simulink model "MdXX_DoneChk"  (R2024b)
settings: Solver=FixedStepDiscrete  StartTime=0.0  StopTime=10.0  FixedStep=0.01  RelTol=1e-3
undefined symbols (not defined in the file or in its folder): KeSMSuVehicleModelConfig_Val
libraries: simulink x44
(part 2 of 3)

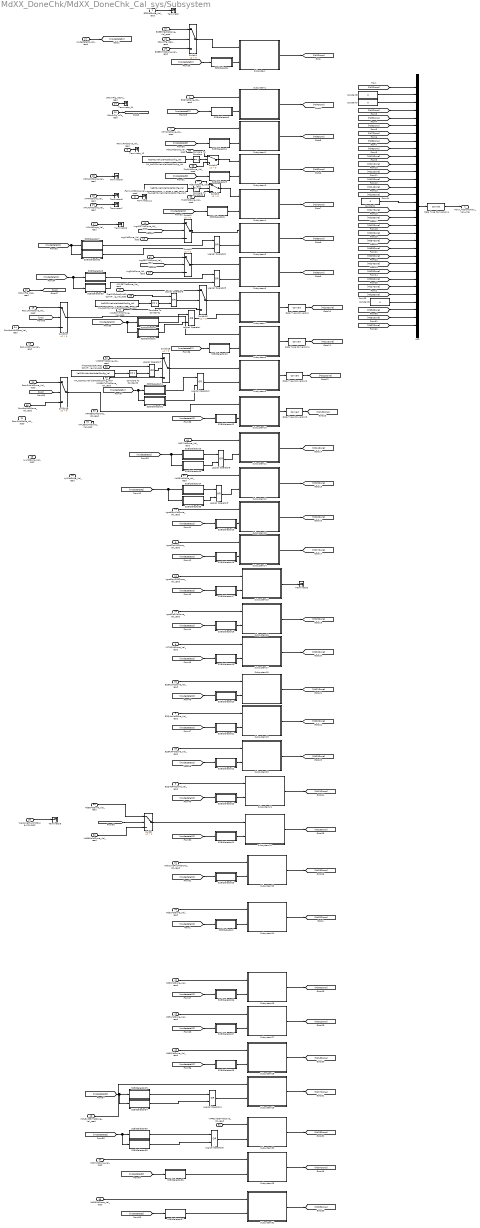
== system MdXX_DoneChk/MdXX_DoneChk_Cal_sys/Subsystem ==
  EZEMdDone_Val_read : Inport
  EZQ4sLMdDone_Val_read : Inport  Port=2
  EZQ4sRMdDone_Val_read : Inport  Port=3
  EZQMdDone_Val_read : Inport  Port=4
  FamlyLMdDone_Val_read : Inport  Port=5
  FamlyRMdDone_Val_read : Inport  Port=6
  INTMLMdDone_Val_read : Inport  Port=7
  INTMRMdDone_Val_read : Inport  Port=8
  LgrstClsLMdDone_Val_read : Inport  Port=9
  LgrstClsRMdDone_Val_read : Inport  Port=10
  LgrstOpnLMdDone_Val_read : Inport  Port=11
  LgrstOpnRMdDone_Val_read : Inport  Port=12
  LugLMdDone_Val_read : Inport  Port=13
  LugRMdDone_Val_read : Inport  Port=14
  LyLMdDone_Val_read : Inport  Port=15
  LyRMdDone_Val_read : Inport  Port=16
  modestate32_Val_read : Inport  Port=17
  RecvL4sMdDone_Val_read : Inport  Port=18
  RecvLMdDone_Val_read : Inport  Port=19
  RecvR4sMdDone_Val_read : Inport  Port=20
  RecvRMdDone_Val_read : Inport  Port=21
  StNumFlg_Is4s_read : Inport  Port=22
  StNumFlg_Is6s_read : Inport  Port=23
  StNumFlg_Is6s7s_read : Inport  Port=24
  StNumFlg_Is7s_read : Inport  Port=25
  VIPL4sMdDone_Val_read : Inport  Port=26
  VIPLMdDone_Val_read : Inport  Port=27
  VIPR4sMdDone_Val_read : Inport  Port=28
  VIPRMdDone_Val_read : Inport  Port=29
  WelcomeBkwdMdDone_Val_read : Inport  Port=30
  WelcomeFwdMdDone_Val_read : Inport  Port=31
  EZE4sLMdDone_Val_read : Inport  Port=32
  EZE4sRMdDone_Val_read : Inport  Port=33
  ComfortMdLDone_Val_read : Inport  Port=34
  ComfortMdRDone_Val_read : Inport  Port=35
  EZE557MdDone_Val_read : Inport  Port=36
  EZE5576sMdDone_Val_read : Inport  Port=37
  IfVeSMSbSecRwLtStCshnFrntUpwdDnwdMovConfig_Val_read : Inport  Port=38
  IfVeSMSbSecRwRtStCshnFrntUpwdDnwdMovConfig_Val_read : Inport  Port=39
  LugL557MdDone_Val_read : Inport  Port=40
  LugR557MdDone_Val_read : Inport  Port=41
  Md30MdDone_Val_read : Inport  Port=42
  Md31MdDone_Val_read : Inport  Port=43
  Md32MdDone_Val_read : Inport  Port=44
  Md53MdDone_Val_read : Inport  Port=45
  VIPL557LTMdDone_Val_read : Inport  Port=46
  VIPL557MdDone_Val_read : Inport  Port=47
  VIPLExit557MdDone_Val_read : Inport  Port=48
  VIPR557LTMdDone_Val_read : Inport  Port=49
  VIPR557MdDone_Val_read : Inport  Port=50
  VIPRExit557MdDone_Val_read : Inport  Port=51
  Md566sMdDone_Val_read : Inport  Port=52
  Md56MdDone_Val_read : Inport  Port=53
  Md57MdDone_Val_read : Inport  Port=54
  Md58MdDone_Val_read : Inport  Port=55
  Md61MdDone_Val_read : Inport  Port=56
  Md62MdDone_Val_read : Inport  Port=57
  FwdLMdDone_Val_read : Inport  Port=58
  FwdRMdDone_Val_read : Inport  Port=59
  Md27MdDone_Val_read : Inport  Port=60
  Md28MdDone_Val_read : Inport  Port=61
  VIPL3582MdDone_Val_read : Inport  Port=62
  VIPR3582MdDone_Val_read : Inport  Port=63
  32BitSelector : Subsystem  mask(32 Bit Selector){BitNum=0}
      mask prompts: BitNum "Select Bit Number"
      mask help: Allows selection of a particular bit (0-31) out of a packed word up to 32 bits long. Output will be true if the bit number selected via the mask parameter is equal to one.
      mask TypeOptions BitNum: 0 | 1 | 2 | 3 | 4 | 5 | 6 | 7 | 8 | 9 | 10 | 11 | 12 | 13 | 14 | 15 | 16 | 17 | 18 | 19 | 20 | 21 | 22 | 23 | 24 | 25 | 26 | 27 | 28 | 29 | 30 | 31
      mask Display:
      | text(0.5, 0.8,'BIT','horizontalAlignment','center')
      | text(0.5, 0.5,'SELECTOR','horizontalAlignment','center')
      | text(0.5, 0.2,['-- Bit ',char(get_param(gcb,'BitNum')),' --'],'horizontalAlignment','center')
  32BitSelector1 : Subsystem  mask(32 Bit Selector){BitNum=31}
      mask prompts: BitNum "Select Bit Number"
      mask help: Allows selection of a particular bit (0-31) out of a packed word up to 32 bits long. Output will be true if the bit number selected via the mask parameter is equal to one.
      mask TypeOptions BitNum: 0 | 1 | 2 | 3 | 4 | 5 | 6 | 7 | 8 | 9 | 10 | 11 | 12 | 13 | 14 | 15 | 16 | 17 | 18 | 19 | 20 | 21 | 22 | 23 | 24 | 25 | 26 | 27 | 28 | 29 | 30 | 31
      mask Display:
      | text(0.5, 0.8,'BIT','horizontalAlignment','center')
      | text(0.5, 0.5,'SELECTOR','horizontalAlignment','center')
      | text(0.5, 0.2,['-- Bit ',char(get_param(gcb,'BitNum')),' --'],'horizontalAlignment','center')
  32BitSelector10 : Subsystem  mask(32 Bit Selector){BitNum=10}
      mask prompts: BitNum "Select Bit Number"
      mask help: Allows selection of a particular bit (0-31) out of a packed word up to 32 bits long. Output will be true if the bit number selected via the mask parameter is equal to one.
      mask TypeOptions BitNum: 0 | 1 | 2 | 3 | 4 | 5 | 6 | 7 | 8 | 9 | 10 | 11 | 12 | 13 | 14 | 15 | 16 | 17 | 18 | 19 | 20 | 21 | 22 | 23 | 24 | 25 | 26 | 27 | 28 | 29 | 30 | 31
      mask Display:
      | text(0.5, 0.8,'BIT','horizontalAlignment','center')
      | text(0.5, 0.5,'SELECTOR','horizontalAlignment','center')
      | text(0.5, 0.2,['-- Bit ',char(get_param(gcb,'BitNum')),' --'],'horizontalAlignment','center')
  32BitSelector11 : Subsystem  mask(32 Bit Selector){BitNum=11}
      mask prompts: BitNum "Select Bit Number"
      mask help: Allows selection of a particular bit (0-31) out of a packed word up to 32 bits long. Output will be true if the bit number selected via the mask parameter is equal to one.
      mask TypeOptions BitNum: 0 | 1 | 2 | 3 | 4 | 5 | 6 | 7 | 8 | 9 | 10 | 11 | 12 | 13 | 14 | 15 | 16 | 17 | 18 | 19 | 20 | 21 | 22 | 23 | 24 | 25 | 26 | 27 | 28 | 29 | 30 | 31
      mask Display:
      | text(0.5, 0.8,'BIT','horizontalAlignment','center')
      | text(0.5, 0.5,'SELECTOR','horizontalAlignment','center')
      | text(0.5, 0.2,['-- Bit ',char(get_param(gcb,'BitNum')),' --'],'horizontalAlignment','center')
  32BitSelector12 : Subsystem  mask(32 Bit Selector){BitNum=12}
      mask prompts: BitNum "Select Bit Number"
      mask help: Allows selection of a particular bit (0-31) out of a packed word up to 32 bits long. Output will be true if the bit number selected via the mask parameter is equal to one.
      mask TypeOptions BitNum: 0 | 1 | 2 | 3 | 4 | 5 | 6 | 7 | 8 | 9 | 10 | 11 | 12 | 13 | 14 | 15 | 16 | 17 | 18 | 19 | 20 | 21 | 22 | 23 | 24 | 25 | 26 | 27 | 28 | 29 | 30 | 31
      mask Display:
      | text(0.5, 0.8,'BIT','horizontalAlignment','center')
      | text(0.5, 0.5,'SELECTOR','horizontalAlignment','center')
      | text(0.5, 0.2,['-- Bit ',char(get_param(gcb,'BitNum')),' --'],'horizontalAlignment','center')
  32BitSelector13 : Subsystem  mask(32 Bit Selector){BitNum=13}
      mask prompts: BitNum "Select Bit Number"
      mask help: Allows selection of a particular bit (0-31) out of a packed word up to 32 bits long. Output will be true if the bit number selected via the mask parameter is equal to one.
      mask TypeOptions BitNum: 0 | 1 | 2 | 3 | 4 | 5 | 6 | 7 | 8 | 9 | 10 | 11 | 12 | 13 | 14 | 15 | 16 | 17 | 18 | 19 | 20 | 21 | 22 | 23 | 24 | 25 | 26 | 27 | 28 | 29 | 30 | 31
      mask Display:
      | text(0.5, 0.8,'BIT','horizontalAlignment','center')
      | text(0.5, 0.5,'SELECTOR','horizontalAlignment','center')
      | text(0.5, 0.2,['-- Bit ',char(get_param(gcb,'BitNum')),' --'],'horizontalAlignment','center')
  32BitSelector14 : Subsystem  mask(32 Bit Selector){BitNum=14}
      mask prompts: BitNum "Select Bit Number"
      mask help: Allows selection of a particular bit (0-31) out of a packed word up to 32 bits long. Output will be true if the bit number selected via the mask parameter is equal to one.
      mask TypeOptions BitNum: 0 | 1 | 2 | 3 | 4 | 5 | 6 | 7 | 8 | 9 | 10 | 11 | 12 | 13 | 14 | 15 | 16 | 17 | 18 | 19 | 20 | 21 | 22 | 23 | 24 | 25 | 26 | 27 | 28 | 29 | 30 | 31
      mask Display:
      | text(0.5, 0.8,'BIT','horizontalAlignment','center')
      | text(0.5, 0.5,'SELECTOR','horizontalAlignment','center')
      | text(0.5, 0.2,['-- Bit ',char(get_param(gcb,'BitNum')),' --'],'horizontalAlignment','center')
  32BitSelector15 : Subsystem  mask(32 Bit Selector){BitNum=15}
      mask prompts: BitNum "Select Bit Number"
      mask help: Allows selection of a particular bit (0-31) out of a packed word up to 32 bits long. Output will be true if the bit number selected via the mask parameter is equal to one.
      mask TypeOptions BitNum: 0 | 1 | 2 | 3 | 4 | 5 | 6 | 7 | 8 | 9 | 10 | 11 | 12 | 13 | 14 | 15 | 16 | 17 | 18 | 19 | 20 | 21 | 22 | 23 | 24 | 25 | 26 | 27 | 28 | 29 | 30 | 31
      mask Display:
      | text(0.5, 0.8,'BIT','horizontalAlignment','center')
      | text(0.5, 0.5,'SELECTOR','horizontalAlignment','center')
      | text(0.5, 0.2,['-- Bit ',char(get_param(gcb,'BitNum')),' --'],'horizontalAlignment','center')
  32BitSelector16 : Subsystem  mask(32 Bit Selector){BitNum=16}
      mask prompts: BitNum "Select Bit Number"
      mask help: Allows selection of a particular bit (0-31) out of a packed word up to 32 bits long. Output will be true if the bit number selected via the mask parameter is equal to one.
      mask TypeOptions BitNum: 0 | 1 | 2 | 3 | 4 | 5 | 6 | 7 | 8 | 9 | 10 | 11 | 12 | 13 | 14 | 15 | 16 | 17 | 18 | 19 | 20 | 21 | 22 | 23 | 24 | 25 | 26 | 27 | 28 | 29 | 30 | 31
      mask Display:
      | text(0.5, 0.8,'BIT','horizontalAlignment','center')
      | text(0.5, 0.5,'SELECTOR','horizontalAlignment','center')
      | text(0.5, 0.2,['-- Bit ',char(get_param(gcb,'BitNum')),' --'],'horizontalAlignment','center')
  32BitSelector17 : Subsystem  mask(32 Bit Selector){BitNum=17}
      mask prompts: BitNum "Select Bit Number"
      mask help: Allows selection of a particular bit (0-31) out of a packed word up to 32 bits long. Output will be true if the bit number selected via the mask parameter is equal to one.
      mask TypeOptions BitNum: 0 | 1 | 2 | 3 | 4 | 5 | 6 | 7 | 8 | 9 | 10 | 11 | 12 | 13 | 14 | 15 | 16 | 17 | 18 | 19 | 20 | 21 | 22 | 23 | 24 | 25 | 26 | 27 | 28 | 29 | 30 | 31
      mask Display:
      | text(0.5, 0.8,'BIT','horizontalAlignment','center')
      | text(0.5, 0.5,'SELECTOR','horizontalAlignment','center')
      | text(0.5, 0.2,['-- Bit ',char(get_param(gcb,'BitNum')),' --'],'horizontalAlignment','center')
  32BitSelector18 : Subsystem  mask(32 Bit Selector){BitNum=18}
      mask prompts: BitNum "Select Bit Number"
      mask help: Allows selection of a particular bit (0-31) out of a packed word up to 32 bits long. Output will be true if the bit number selected via the mask parameter is equal to one.
      mask TypeOptions BitNum: 0 | 1 | 2 | 3 | 4 | 5 | 6 | 7 | 8 | 9 | 10 | 11 | 12 | 13 | 14 | 15 | 16 | 17 | 18 | 19 | 20 | 21 | 22 | 23 | 24 | 25 | 26 | 27 | 28 | 29 | 30 | 31
      mask Display:
      | text(0.5, 0.8,'BIT','horizontalAlignment','center')
      | text(0.5, 0.5,'SELECTOR','horizontalAlignment','center')
      | text(0.5, 0.2,['-- Bit ',char(get_param(gcb,'BitNum')),' --'],'horizontalAlignment','center')
  32BitSelector19 : Subsystem  mask(32 Bit Selector){BitNum=19}
      mask prompts: BitNum "Select Bit Number"
      mask help: Allows selection of a particular bit (0-31) out of a packed word up to 32 bits long. Output will be true if the bit number selected via the mask parameter is equal to one.
      mask TypeOptions BitNum: 0 | 1 | 2 | 3 | 4 | 5 | 6 | 7 | 8 | 9 | 10 | 11 | 12 | 13 | 14 | 15 | 16 | 17 | 18 | 19 | 20 | 21 | 22 | 23 | 24 | 25 | 26 | 27 | 28 | 29 | 30 | 31
      mask Display:
      | text(0.5, 0.8,'BIT','horizontalAlignment','center')
      | text(0.5, 0.5,'SELECTOR','horizontalAlignment','center')
      | text(0.5, 0.2,['-- Bit ',char(get_param(gcb,'BitNum')),' --'],'horizontalAlignment','center')
  32BitSelector2 : Subsystem  mask(32 Bit Selector){BitNum=1}
      mask prompts: BitNum "Select Bit Number"
      mask help: Allows selection of a particular bit (0-31) out of a packed word up to 32 bits long. Output will be true if the bit number selected via the mask parameter is equal to one.
      mask TypeOptions BitNum: 0 | 1 | 2 | 3 | 4 | 5 | 6 | 7 | 8 | 9 | 10 | 11 | 12 | 13 | 14 | 15 | 16 | 17 | 18 | 19 | 20 | 21 | 22 | 23 | 24 | 25 | 26 | 27 | 28 | 29 | 30 | 31
      mask Display:
      | text(0.5, 0.8,'BIT','horizontalAlignment','center')
      | text(0.5, 0.5,'SELECTOR','horizontalAlignment','center')
      | text(0.5, 0.2,['-- Bit ',char(get_param(gcb,'BitNum')),' --'],'horizontalAlignment','center')
  32BitSelector20 : Subsystem  mask(32 Bit Selector){BitNum=20}
      mask prompts: BitNum "Select Bit Number"
      mask help: Allows selection of a particular bit (0-31) out of a packed word up to 32 bits long. Output will be true if the bit number selected via the mask parameter is equal to one.
      mask TypeOptions BitNum: 0 | 1 | 2 | 3 | 4 | 5 | 6 | 7 | 8 | 9 | 10 | 11 | 12 | 13 | 14 | 15 | 16 | 17 | 18 | 19 | 20 | 21 | 22 | 23 | 24 | 25 | 26 | 27 | 28 | 29 | 30 | 31
      mask Display:
      | text(0.5, 0.8,'BIT','horizontalAlignment','center')
      | text(0.5, 0.5,'SELECTOR','horizontalAlignment','center')
      | text(0.5, 0.2,['-- Bit ',char(get_param(gcb,'BitNum')),' --'],'horizontalAlignment','center')
  32BitSelector21 : Subsystem  mask(32 Bit Selector){BitNum=21}
      mask prompts: BitNum "Select Bit Number"
      mask help: Allows selection of a particular bit (0-31) out of a packed word up to 32 bits long. Output will be true if the bit number selected via the mask parameter is equal to one.
      mask TypeOptions BitNum: 0 | 1 | 2 | 3 | 4 | 5 | 6 | 7 | 8 | 9 | 10 | 11 | 12 | 13 | 14 | 15 | 16 | 17 | 18 | 19 | 20 | 21 | 22 | 23 | 24 | 25 | 26 | 27 | 28 | 29 | 30 | 31
      mask Display:
      | text(0.5, 0.8,'BIT','horizontalAlignment','center')
      | text(0.5, 0.5,'SELECTOR','horizontalAlignment','center')
      | text(0.5, 0.2,['-- Bit ',char(get_param(gcb,'BitNum')),' --'],'horizontalAlignment','center')
  32BitSelector22 : Subsystem  mask(32 Bit Selector){BitNum=22}
      mask prompts: BitNum "Select Bit Number"
      mask help: Allows selection of a particular bit (0-31) out of a packed word up to 32 bits long. Output will be true if the bit number selected via the mask parameter is equal to one.
      mask TypeOptions BitNum: 0 | 1 | 2 | 3 | 4 | 5 | 6 | 7 | 8 | 9 | 10 | 11 | 12 | 13 | 14 | 15 | 16 | 17 | 18 | 19 | 20 | 21 | 22 | 23 | 24 | 25 | 26 | 27 | 28 | 29 | 30 | 31
      mask Display:
      | text(0.5, 0.8,'BIT','horizontalAlignment','center')
      | text(0.5, 0.5,'SELECTOR','horizontalAlignment','center')
      | text(0.5, 0.2,['-- Bit ',char(get_param(gcb,'BitNum')),' --'],'horizontalAlignment','center')
  32BitSelector23 : Subsystem  mask(32 Bit Selector){BitNum=23}
      mask prompts: BitNum "Select Bit Number"
      mask help: Allows selection of a particular bit (0-31) out of a packed word up to 32 bits long. Output will be true if the bit number selected via the mask parameter is equal to one.
      mask TypeOptions BitNum: 0 | 1 | 2 | 3 | 4 | 5 | 6 | 7 | 8 | 9 | 10 | 11 | 12 | 13 | 14 | 15 | 16 | 17 | 18 | 19 | 20 | 21 | 22 | 23 | 24 | 25 | 26 | 27 | 28 | 29 | 30 | 31
      mask Display:
      | text(0.5, 0.8,'BIT','horizontalAlignment','center')
      | text(0.5, 0.5,'SELECTOR','horizontalAlignment','center')
      | text(0.5, 0.2,['-- Bit ',char(get_param(gcb,'BitNum')),' --'],'horizontalAlignment','center')
  32BitSelector24 : Subsystem  mask(32 Bit Selector){BitNum=24}
      mask prompts: BitNum "Select Bit Number"
      mask help: Allows selection of a particular bit (0-31) out of a packed word up to 32 bits long. Output will be true if the bit number selected via the mask parameter is equal to one.
      mask TypeOptions BitNum: 0 | 1 | 2 | 3 | 4 | 5 | 6 | 7 | 8 | 9 | 10 | 11 | 12 | 13 | 14 | 15 | 16 | 17 | 18 | 19 | 20 | 21 | 22 | 23 | 24 | 25 | 26 | 27 | 28 | 29 | 30 | 31
      mask Display:
      | text(0.5, 0.8,'BIT','horizontalAlignment','center')
      | text(0.5, 0.5,'SELECTOR','horizontalAlignment','center')
      | text(0.5, 0.2,['-- Bit ',char(get_param(gcb,'BitNum')),' --'],'horizontalAlignment','center')
  32BitSelector25 : Subsystem  mask(32 Bit Selector){BitNum=25}
      mask prompts: BitNum "Select Bit Number"
      mask help: Allows selection of a particular bit (0-31) out of a packed word up to 32 bits long. Output will be true if the bit number selected via the mask parameter is equal to one.
      mask TypeOptions BitNum: 0 | 1 | 2 | 3 | 4 | 5 | 6 | 7 | 8 | 9 | 10 | 11 | 12 | 13 | 14 | 15 | 16 | 17 | 18 | 19 | 20 | 21 | 22 | 23 | 24 | 25 | 26 | 27 | 28 | 29 | 30 | 31
      mask Display:
      | text(0.5, 0.8,'BIT','horizontalAlignment','center')
      | text(0.5, 0.5,'SELECTOR','horizontalAlignment','center')
      | text(0.5, 0.2,['-- Bit ',char(get_param(gcb,'BitNum')),' --'],'horizontalAlignment','center')
  32BitSelector26 : Subsystem  mask(32 Bit Selector){BitNum=29}
      mask prompts: BitNum "Select Bit Number"
      mask help: Allows selection of a particular bit (0-31) out of a packed word up to 32 bits long. Output will be true if the bit number selected via the mask parameter is equal to one.
      mask TypeOptions BitNum: 0 | 1 | 2 | 3 | 4 | 5 | 6 | 7 | 8 | 9 | 10 | 11 | 12 | 13 | 14 | 15 | 16 | 17 | 18 | 19 | 20 | 21 | 22 | 23 | 24 | 25 | 26 | 27 | 28 | 29 | 30 | 31
      mask Display:
      | text(0.5, 0.8,'BIT','horizontalAlignment','center')
      | text(0.5, 0.5,'SELECTOR','horizontalAlignment','center')
      | text(0.5, 0.2,['-- Bit ',char(get_param(gcb,'BitNum')),' --'],'horizontalAlignment','center')
  32BitSelector27 : Subsystem  mask(32 Bit Selector){BitNum=30}
      mask prompts: BitNum "Select Bit Number"
      mask help: Allows selection of a particular bit (0-31) out of a packed word up to 32 bits long. Output will be true if the bit number selected via the mask parameter is equal to one.
      mask TypeOptions BitNum: 0 | 1 | 2 | 3 | 4 | 5 | 6 | 7 | 8 | 9 | 10 | 11 | 12 | 13 | 14 | 15 | 16 | 17 | 18 | 19 | 20 | 21 | 22 | 23 | 24 | 25 | 26 | 27 | 28 | 29 | 30 | 31
      mask Display:
      | text(0.5, 0.8,'BIT','horizontalAlignment','center')
      | text(0.5, 0.5,'SELECTOR','horizontalAlignment','center')
      | text(0.5, 0.2,['-- Bit ',char(get_param(gcb,'BitNum')),' --'],'horizontalAlignment','center')
  32BitSelector28 : Subsystem  mask(32 Bit Selector){BitNum=17}
      mask prompts: BitNum "Select Bit Number"
      mask help: Allows selection of a particular bit (0-31) out of a packed word up to 32 bits long. Output will be true if the bit number selected via the mask parameter is equal to one.
      mask TypeOptions BitNum: 0 | 1 | 2 | 3 | 4 | 5 | 6 | 7 | 8 | 9 | 10 | 11 | 12 | 13 | 14 | 15 | 16 | 17 | 18 | 19 | 20 | 21 | 22 | 23 | 24 | 25 | 26 | 27 | 28 | 29 | 30 | 31
      mask Display:
      | text(0.5, 0.8,'BIT','horizontalAlignment','center')
      | text(0.5, 0.5,'SELECTOR','horizontalAlignment','center')
      | text(0.5, 0.2,['-- Bit ',char(get_param(gcb,'BitNum')),' --'],'horizontalAlignment','center')
  32BitSelector29 : Subsystem  mask(32 Bit Selector){BitNum=26}
      mask prompts: BitNum "Select Bit Number"
      mask help: Allows selection of a particular bit (0-31) out of a packed word up to 32 bits long. Output will be true if the bit number selected via the mask parameter is equal to one.
      mask TypeOptions BitNum: 0 | 1 | 2 | 3 | 4 | 5 | 6 | 7 | 8 | 9 | 10 | 11 | 12 | 13 | 14 | 15 | 16 | 17 | 18 | 19 | 20 | 21 | 22 | 23 | 24 | 25 | 26 | 27 | 28 | 29 | 30 | 31
      mask Display:
      | text(0.5, 0.8,'BIT','horizontalAlignment','center')
      | text(0.5, 0.5,'SELECTOR','horizontalAlignment','center')
      | text(0.5, 0.2,['-- Bit ',char(get_param(gcb,'BitNum')),' --'],'horizontalAlignment','center')
  32BitSelector3 : Subsystem  mask(32 Bit Selector){BitNum=3}
      mask prompts: BitNum "Select Bit Number"
      mask help: Allows selection of a particular bit (0-31) out of a packed word up to 32 bits long. Output will be true if the bit number selected via the mask parameter is equal to one.
      mask TypeOptions BitNum: 0 | 1 | 2 | 3 | 4 | 5 | 6 | 7 | 8 | 9 | 10 | 11 | 12 | 13 | 14 | 15 | 16 | 17 | 18 | 19 | 20 | 21 | 22 | 23 | 24 | 25 | 26 | 27 | 28 | 29 | 30 | 31
      mask Display:
      | text(0.5, 0.8,'BIT','horizontalAlignment','center')
      | text(0.5, 0.5,'SELECTOR','horizontalAlignment','center')
      | text(0.5, 0.2,['-- Bit ',char(get_param(gcb,'BitNum')),' --'],'horizontalAlignment','center')
  32BitSelector30 : Subsystem  mask(32 Bit Selector){BitNum=27}
      mask prompts: BitNum "Select Bit Number"
      mask help: Allows selection of a particular bit (0-31) out of a packed word up to 32 bits long. Output will be true if the bit number selected via the mask parameter is equal to one.
      mask TypeOptions BitNum: 0 | 1 | 2 | 3 | 4 | 5 | 6 | 7 | 8 | 9 | 10 | 11 | 12 | 13 | 14 | 15 | 16 | 17 | 18 | 19 | 20 | 21 | 22 | 23 | 24 | 25 | 26 | 27 | 28 | 29 | 30 | 31
      mask Display:
      | text(0.5, 0.8,'BIT','horizontalAlignment','center')
      | text(0.5, 0.5,'SELECTOR','horizontalAlignment','center')
      | text(0.5, 0.2,['-- Bit ',char(get_param(gcb,'BitNum')),' --'],'horizontalAlignment','center')
  32BitSelector31 : Subsystem  mask(32 Bit Selector){BitNum=1}
      mask prompts: BitNum "Select Bit Number"
      mask help: Allows selection of a particular bit (0-31) out of a packed word up to 32 bits long. Output will be true if the bit number selected via the mask parameter is equal to one.
      mask TypeOptions BitNum: 0 | 1 | 2 | 3 | 4 | 5 | 6 | 7 | 8 | 9 | 10 | 11 | 12 | 13 | 14 | 15 | 16 | 17 | 18 | 19 | 20 | 21 | 22 | 23 | 24 | 25 | 26 | 27 | 28 | 29 | 30 | 31
      mask Display:
      | text(0.5, 0.8,'BIT','horizontalAlignment','center')
      | text(0.5, 0.5,'SELECTOR','horizontalAlignment','center')
      | text(0.5, 0.2,['-- Bit ',char(get_param(gcb,'BitNum')),' --'],'horizontalAlignment','center')
  32BitSelector32 : Subsystem  mask(32 Bit Selector){BitNum=2}
      mask prompts: BitNum "Select Bit Number"
      mask help: Allows selection of a particular bit (0-31) out of a packed word up to 32 bits long. Output will be true if the bit number selected via the mask parameter is equal to one.
      mask TypeOptions BitNum: 0 | 1 | 2 | 3 | 4 | 5 | 6 | 7 | 8 | 9 | 10 | 11 | 12 | 13 | 14 | 15 | 16 | 17 | 18 | 19 | 20 | 21 | 22 | 23 | 24 | 25 | 26 | 27 | 28 | 29 | 30 | 31
      mask Display:
      | text(0.5, 0.8,'BIT','horizontalAlignment','center')
      | text(0.5, 0.5,'SELECTOR','horizontalAlignment','center')
      | text(0.5, 0.2,['-- Bit ',char(get_param(gcb,'BitNum')),' --'],'horizontalAlignment','center')
  32BitSelector33 : Subsystem  mask(32 Bit Selector){BitNum=2}
      mask prompts: BitNum "Select Bit Number"
      mask help: Allows selection of a particular bit (0-31) out of a packed word up to 32 bits long. Output will be true if the bit number selected via the mask parameter is equal to one.
      mask TypeOptions BitNum: 0 | 1 | 2 | 3 | 4 | 5 | 6 | 7 | 8 | 9 | 10 | 11 | 12 | 13 | 14 | 15 | 16 | 17 | 18 | 19 | 20 | 21 | 22 | 23 | 24 | 25 | 26 | 27 | 28 | 29 | 30 | 31
      mask Display:
      | text(0.5, 0.8,'BIT','horizontalAlignment','center')
      | text(0.5, 0.5,'SELECTOR','horizontalAlignment','center')
      | text(0.5, 0.2,['-- Bit ',char(get_param(gcb,'BitNum')),' --'],'horizontalAlignment','center')
  32BitSelector34 : Subsystem  mask(32 Bit Selector){BitNum=28}
      mask prompts: BitNum "Select Bit Number"
      mask help: Allows selection of a particular bit (0-31) out of a packed word up to 32 bits long. Output will be true if the bit number selected via the mask parameter is equal to one.
      mask TypeOptions BitNum: 0 | 1 | 2 | 3 | 4 | 5 | 6 | 7 | 8 | 9 | 10 | 11 | 12 | 13 | 14 | 15 | 16 | 17 | 18 | 19 | 20 | 21 | 22 | 23 | 24 | 25 | 26 | 27 | 28 | 29 | 30 | 31
      mask Display:
      | text(0.5, 0.8,'BIT','horizontalAlignment','center')
      | text(0.5, 0.5,'SELECTOR','horizontalAlignment','center')
      | text(0.5, 0.2,['-- Bit ',char(get_param(gcb,'BitNum')),' --'],'horizontalAlignment','center')
  32BitSelector35 : Subsystem  mask(32 Bit Selector){BitNum=28}
      mask prompts: BitNum "Select Bit Number"
      mask help: Allows selection of a particular bit (0-31) out of a packed word up to 32 bits long. Output will be true if the bit number selected via the mask parameter is equal to one.
      mask TypeOptions BitNum: 0 | 1 | 2 | 3 | 4 | 5 | 6 | 7 | 8 | 9 | 10 | 11 | 12 | 13 | 14 | 15 | 16 | 17 | 18 | 19 | 20 | 21 | 22 | 23 | 24 | 25 | 26 | 27 | 28 | 29 | 30 | 31
      mask Display:
      | text(0.5, 0.8,'BIT','horizontalAlignment','center')
      | text(0.5, 0.5,'SELECTOR','horizontalAlignment','center')
      | text(0.5, 0.2,['-- Bit ',char(get_param(gcb,'BitNum')),' --'],'horizontalAlignment','center')
  32BitSelector36 : Subsystem  mask(32 Bit Selector){BitNum=20}
      mask prompts: BitNum "Select Bit Number"
      mask help: Allows selection of a particular bit (0-31) out of a packed word up to 32 bits long. Output will be true if the bit number selected via the mask parameter is equal to one.
      mask TypeOptions BitNum: 0 | 1 | 2 | 3 | 4 | 5 | 6 | 7 | 8 | 9 | 10 | 11 | 12 | 13 | 14 | 15 | 16 | 17 | 18 | 19 | 20 | 21 | 22 | 23 | 24 | 25 | 26 | 27 | 28 | 29 | 30 | 31
      mask Display:
      | text(0.5, 0.8,'BIT','horizontalAlignment','center')
      | text(0.5, 0.5,'SELECTOR','horizontalAlignment','center')
      | text(0.5, 0.2,['-- Bit ',char(get_param(gcb,'BitNum')),' --'],'horizontalAlignment','center')
  32BitSelector37 : Subsystem  mask(32 Bit Selector){BitNum=21}
      mask prompts: BitNum "Select Bit Number"
      mask help: Allows selection of a particular bit (0-31) out of a packed word up to 32 bits long. Output will be true if the bit number selected via the mask parameter is equal to one.
      mask TypeOptions BitNum: 0 | 1 | 2 | 3 | 4 | 5 | 6 | 7 | 8 | 9 | 10 | 11 | 12 | 13 | 14 | 15 | 16 | 17 | 18 | 19 | 20 | 21 | 22 | 23 | 24 | 25 | 26 | 27 | 28 | 29 | 30 | 31
      mask Display:
      | text(0.5, 0.8,'BIT','horizontalAlignment','center')
      | text(0.5, 0.5,'SELECTOR','horizontalAlignment','center')
      | text(0.5, 0.2,['-- Bit ',char(get_param(gcb,'BitNum')),' --'],'horizontalAlignment','center')
  32BitSelector38 : Subsystem  mask(32 Bit Selector){BitNum=15}
      mask prompts: BitNum "Select Bit Number"
      mask help: Allows selection of a particular bit (0-31) out of a packed word up to 32 bits long. Output will be true if the bit number selected via the mask parameter is equal to one.
      mask TypeOptions BitNum: 0 | 1 | 2 | 3 | 4 | 5 | 6 | 7 | 8 | 9 | 10 | 11 | 12 | 13 | 14 | 15 | 16 | 17 | 18 | 19 | 20 | 21 | 22 | 23 | 24 | 25 | 26 | 27 | 28 | 29 | 30 | 31
      mask Display:
      | text(0.5, 0.8,'BIT','horizontalAlignment','center')
      | text(0.5, 0.5,'SELECTOR','horizontalAlignment','center')
      | text(0.5, 0.2,['-- Bit ',char(get_param(gcb,'BitNum')),' --'],'horizontalAlignment','center')
  32BitSelector39 : Subsystem  mask(32 Bit Selector){BitNum=15}
      mask prompts: BitNum "Select Bit Number"
      mask help: Allows selection of a particular bit (0-31) out of a packed word up to 32 bits long. Output will be true if the bit number selected via the mask parameter is equal to one.
      mask TypeOptions BitNum: 0 | 1 | 2 | 3 | 4 | 5 | 6 | 7 | 8 | 9 | 10 | 11 | 12 | 13 | 14 | 15 | 16 | 17 | 18 | 19 | 20 | 21 | 22 | 23 | 24 | 25 | 26 | 27 | 28 | 29 | 30 | 31
      mask Display:
      | text(0.5, 0.8,'BIT','horizontalAlignment','center')
      | text(0.5, 0.5,'SELECTOR','horizontalAlignment','center')
      | text(0.5, 0.2,['-- Bit ',char(get_param(gcb,'BitNum')),' --'],'horizontalAlignment','center')
  32BitSelector4 : Subsystem  mask(32 Bit Selector){BitNum=4}
      mask prompts: BitNum "Select Bit Number"
      mask help: Allows selection of a particular bit (0-31) out of a packed word up to 32 bits long. Output will be true if the bit number selected via the mask parameter is equal to one.
      mask TypeOptions BitNum: 0 | 1 | 2 | 3 | 4 | 5 | 6 | 7 | 8 | 9 | 10 | 11 | 12 | 13 | 14 | 15 | 16 | 17 | 18 | 19 | 20 | 21 | 22 | 23 | 24 | 25 | 26 | 27 | 28 | 29 | 30 | 31
      mask Display:
      | text(0.5, 0.8,'BIT','horizontalAlignment','center')
      | text(0.5, 0.5,'SELECTOR','horizontalAlignment','center')
      | text(0.5, 0.2,['-- Bit ',char(get_param(gcb,'BitNum')),' --'],'horizontalAlignment','center')
  32BitSelector5 : Subsystem  mask(32 Bit Selector){BitNum=5}
      mask prompts: BitNum "Select Bit Number"
      mask help: Allows selection of a particular bit (0-31) out of a packed word up to 32 bits long. Output will be true if the bit number selected via the mask parameter is equal to one.
      mask TypeOptions BitNum: 0 | 1 | 2 | 3 | 4 | 5 | 6 | 7 | 8 | 9 | 10 | 11 | 12 | 13 | 14 | 15 | 16 | 17 | 18 | 19 | 20 | 21 | 22 | 23 | 24 | 25 | 26 | 27 | 28 | 29 | 30 | 31
      mask Display:
      | text(0.5, 0.8,'BIT','horizontalAlignment','center')
      | text(0.5, 0.5,'SELECTOR','horizontalAlignment','center')
      | text(0.5, 0.2,['-- Bit ',char(get_param(gcb,'BitNum')),' --'],'horizontalAlignment','center')
  32BitSelector6 : Subsystem  mask(32 Bit Selector){BitNum=6}
      mask prompts: BitNum "Select Bit Number"
      mask help: Allows selection of a particular bit (0-31) out of a packed word up to 32 bits long. Output will be true if the bit number selected via the mask parameter is equal to one.
      mask TypeOptions BitNum: 0 | 1 | 2 | 3 | 4 | 5 | 6 | 7 | 8 | 9 | 10 | 11 | 12 | 13 | 14 | 15 | 16 | 17 | 18 | 19 | 20 | 21 | 22 | 23 | 24 | 25 | 26 | 27 | 28 | 29 | 30 | 31
      mask Display:
      | text(0.5, 0.8,'BIT','horizontalAlignment','center')
      | text(0.5, 0.5,'SELECTOR','horizontalAlignment','center')
      | text(0.5, 0.2,['-- Bit ',char(get_param(gcb,'BitNum')),' --'],'horizontalAlignment','center')
  32BitSelector7 : Subsystem  mask(32 Bit Selector){BitNum=7}
      mask prompts: BitNum "Select Bit Number"
      mask help: Allows selection of a particular bit (0-31) out of a packed word up to 32 bits long. Output will be true if the bit number selected via the mask parameter is equal to one.
      mask TypeOptions BitNum: 0 | 1 | 2 | 3 | 4 | 5 | 6 | 7 | 8 | 9 | 10 | 11 | 12 | 13 | 14 | 15 | 16 | 17 | 18 | 19 | 20 | 21 | 22 | 23 | 24 | 25 | 26 | 27 | 28 | 29 | 30 | 31
      mask Display:
      | text(0.5, 0.8,'BIT','horizontalAlignment','center')
      | text(0.5, 0.5,'SELECTOR','horizontalAlignment','center')
      | text(0.5, 0.2,['-- Bit ',char(get_param(gcb,'BitNum')),' --'],'horizontalAlignment','center')
  32BitSelector8 : Subsystem  mask(32 Bit Selector){BitNum=8}
      mask prompts: BitNum "Select Bit Number"
      mask help: Allows selection of a particular bit (0-31) out of a packed word up to 32 bits long. Output will be true if the bit number selected via the mask parameter is equal to one.
      mask TypeOptions BitNum: 0 | 1 | 2 | 3 | 4 | 5 | 6 | 7 | 8 | 9 | 10 | 11 | 12 | 13 | 14 | 15 | 16 | 17 | 18 | 19 | 20 | 21 | 22 | 23 | 24 | 25 | 26 | 27 | 28 | 29 | 30 | 31
      mask Display:
      | text(0.5, 0.8,'BIT','horizontalAlignment','center')
      | text(0.5, 0.5,'SELECTOR','horizontalAlignment','center')
      | text(0.5, 0.2,['-- Bit ',char(get_param(gcb,'BitNum')),' --'],'horizontalAlignment','center')
  32BitSelector9 : Subsystem  mask(32 Bit Selector){BitNum=9}
      mask prompts: BitNum "Select Bit Number"
      mask help: Allows selection of a particular bit (0-31) out of a packed word up to 32 bits long. Output will be true if the bit number selected via the mask parameter is equal to one.
      mask TypeOptions BitNum: 0 | 1 | 2 | 3 | 4 | 5 | 6 | 7 | 8 | 9 | 10 | 11 | 12 | 13 | 14 | 15 | 16 | 17 | 18 | 19 | 20 | 21 | 22 | 23 | 24 | 25 | 26 | 27 | 28 | 29 | 30 | 31
      mask Display:
      | text(0.5, 0.8,'BIT','horizontalAlignment','center')
      | text(0.5, 0.5,'SELECTOR','horizontalAlignment','center')
      | text(0.5, 0.2,['-- Bit ',char(get_param(gcb,'BitNum')),' --'],'horizontalAlignment','center')
  Compare To Constant{,1..3} (4 alike) : simulink/Logic and Bit Operations/Compare To Constant  relop===  const=1  OutDataTypeStr=boolean
  Constant{1,3,7..8} (4 alike) : Constant  Value=0  OutDataTypeStr=uint8
  Data Type Conversion{,1..4} (5 alike) : DataTypeConversion  SaturateOnIntegerOverflow=off  RndMeth=Floor
  Logical Operator{,1..9} (10 alike) : Logic  Operator=OR  AllPortsSameDT=off  OutDataTypeStr=boolean
  Mux : Mux  Inputs=32
  PA_KeSMSuVehicleModelConfig_Val{,1..3} (4 alike) : Constant  Value=KeSMSuVehicleModelConfig_Val
  Subsystem : Subsystem  TreatAsAtomicUnit=on  RTWFcnName=MdDoneSelc
      settings: RTWFcnNameOpts=User specified
  Subsystem1 : Subsystem  TreatAsAtomicUnit=on  RTWFcnName=MdDoneSelc
      settings: RTWFcnNameOpts=User specified
  Subsystem10 : Subsystem  TreatAsAtomicUnit=on  RTWFcnName=MdDoneSelc
      settings: RTWFcnNameOpts=User specified
  Subsystem11 : Subsystem  TreatAsAtomicUnit=on  RTWFcnName=MdDoneSelc
      settings: RTWFcnNameOpts=User specified
  Subsystem12 : Subsystem  TreatAsAtomicUnit=on  RTWFcnName=MdDoneSelc
      settings: RTWFcnNameOpts=User specified
  Subsystem13 : Subsystem  TreatAsAtomicUnit=on  RTWFcnName=MdDoneSelc
      settings: RTWFcnNameOpts=User specified
  Subsystem14 : Subsystem  TreatAsAtomicUnit=on  RTWFcnName=MdDoneSelc
      settings: RTWFcnNameOpts=User specified
  Subsystem15 : Subsystem  TreatAsAtomicUnit=on  RTWFcnName=MdDoneSelc
      settings: RTWFcnNameOpts=User specified
  Subsystem16 : Subsystem  TreatAsAtomicUnit=on  RTWFcnName=MdDoneSelc
      settings: RTWFcnNameOpts=User specified
  Subsystem17 : Subsystem  TreatAsAtomicUnit=on  RTWFcnName=MdDoneSelc
      settings: RTWFcnNameOpts=User specified
  Subsystem18 : Subsystem  TreatAsAtomicUnit=on  RTWFcnName=MdDoneSelc
      settings: RTWFcnNameOpts=User specified
  Subsystem19 : Subsystem  TreatAsAtomicUnit=on  RTWFcnName=MdDoneSelc
      settings: RTWFcnNameOpts=User specified
  Subsystem2 : Subsystem  TreatAsAtomicUnit=on  RTWFcnName=MdDoneSelc
      settings: RTWFcnNameOpts=User specified
  Subsystem20 : Subsystem  TreatAsAtomicUnit=on  RTWFcnName=MdDoneSelc
      settings: RTWFcnNameOpts=User specified
  Subsystem21 : Subsystem  TreatAsAtomicUnit=on  RTWFcnName=MdDoneSelc
      settings: RTWFcnNameOpts=User specified
  Subsystem22 : Subsystem  TreatAsAtomicUnit=on  RTWFcnName=MdDoneSelc
      settings: RTWFcnNameOpts=User specified
  Subsystem23 : Subsystem  TreatAsAtomicUnit=on  RTWFcnName=MdDoneSelc
      settings: RTWFcnNameOpts=User specified
  Subsystem24 : Subsystem  TreatAsAtomicUnit=on  RTWFcnName=MdDoneSelc
      settings: RTWFcnNameOpts=User specified
  Subsystem25 : Subsystem  TreatAsAtomicUnit=on  RTWFcnName=MdDoneSelc
      settings: RTWFcnNameOpts=User specified
  Subsystem26 : Subsystem  TreatAsAtomicUnit=on  RTWFcnName=MdDoneSelc
      settings: RTWFcnNameOpts=User specified
  Subsystem27 : Subsystem  TreatAsAtomicUnit=on  RTWFcnName=MdDoneSelc
      settings: RTWFcnNameOpts=User specified
  Subsystem28 : Subsystem  TreatAsAtomicUnit=on  RTWFcnName=MdDoneSelc
      settings: RTWFcnNameOpts=User specified
  Subsystem29 : Subsystem  TreatAsAtomicUnit=on  RTWFcnName=MdDoneSelc
      settings: RTWFcnNameOpts=User specified
  Subsystem3 : Subsystem  TreatAsAtomicUnit=on  RTWFcnName=MdDoneSelc
      settings: RTWFcnNameOpts=User specified
  Subsystem30 : Subsystem  TreatAsAtomicUnit=on  RTWFcnName=MdDoneSelc
      settings: RTWFcnNameOpts=User specified
  Subsystem31 : Subsystem  TreatAsAtomicUnit=on  RTWFcnName=MdDoneSelc
      settings: RTWFcnNameOpts=User specified
  Subsystem4 : Subsystem  TreatAsAtomicUnit=on  RTWFcnName=MdDoneSelc
      settings: RTWFcnNameOpts=User specified
  Subsystem5 : Subsystem  TreatAsAtomicUnit=on  RTWFcnName=MdDoneSelc
      settings: RTWFcnNameOpts=User specified
  Subsystem6 : Subsystem  TreatAsAtomicUnit=on  RTWFcnName=MdDoneSelc
      settings: RTWFcnNameOpts=User specified
  Subsystem7 : Subsystem  TreatAsAtomicUnit=on  RTWFcnName=MdDoneSelc
      settings: RTWFcnNameOpts=User specified
  Subsystem8 : Subsystem  TreatAsAtomicUnit=on  RTWFcnName=MdDoneSelc
      settings: RTWFcnNameOpts=User specified
  Subsystem9 : Subsystem  TreatAsAtomicUnit=on  RTWFcnName=MdDoneSelc
      settings: RTWFcnNameOpts=User specified
  Switch{,1..5,26..29} (10 alike) : Switch  Criteria=u2 > Threshold  SaturateOnIntegerOverflow=off  InputSameDT=off
  Terminator{,3,5..9} (7 alike) : Terminator
  Terminator_11 : Terminator
  Terminator_12 : Terminator
  Terminator_24 : Terminator
  MdXX_MdDoneArray_Val_write : Outport  VectorParamsAs1DForOutWhenUnconnected=off
      settings: EnsureOutportIsVirtual=on
  wires:
  StNumFlg_Is7s_read/1 -> [is7s]
  StNumFlg_Is6s_read/1 -> Switch1/2
  StNumFlg_Is6s7s_read/1 -> Terminator_24/1
  StNumFlg_Is4s_read/1 -> [is4s]
  Mux/1 -> Data Type Conversion4/1
  [Md1Done] -> Mux/1
  Constant8/1 -> Mux/2
  Constant7/1 -> Mux/3
  [Md4Done] -> Mux/4
  [Md5Done] -> Mux/5
  [Md6Done] -> Mux/6
  [Md7Done] -> Mux/7
  [Md8Done] -> Mux/8
  [Md9Done] -> Mux/9
  [Md10Done] -> Mux/10
  [Md20Done] -> Mux/20
  [Md19Done] -> Mux/19
  [Md18Done] -> Mux/18
  [Md17Done] -> Mux/17
  Constant1/1 -> Mux/16
  [Md15Done] -> Mux/15
  [Md14Done] -> Mux/14
  [Md13Done] -> Mux/13
  [Md12Done] -> Mux/12
  [Md11Done] -> Mux/11
  [Md30Done] -> Mux/30
  Constant3/1 -> Mux/29
  [Md28Done] -> Mux/28
  [Md27Done] -> Mux/27
  [Md26Done] -> Mux/26
  [Md25Done] -> Mux/25
  [Md24Done] -> Mux/24
  [Md23Done] -> Mux/23
  [Md58Done] -> Mux/22
  [Md57Done] -> Mux/21
  [Md31Done] -> Mux/31
  [Md32Done] -> Mux/32
  modestate32_Val_read/1 -> [modestate32]
  [modestate32] -> 32BitSelector3/1(x)
  [modestate32] -> 32BitSelector4/1(x)
  [modestate32] -> 32BitSelector5/1(x)
  Subsystem4/1(MdDoneOut) -> [Md7Done]
  [modestate32] -> 32BitSelector6/1(x)
  [modestate32] -> 32BitSelector32/1(x), 32BitSelector7/1(x)
  [modestate32] -> 32BitSelector2/1(x), 32BitSelector9/1(x)
  [modestate32] -> 32BitSelector10/1(x)
  [modestate32] -> 32BitSelector31/1(x), 32BitSelector11/1(x)
  [modestate32] -> 32BitSelector12/1(x)
  [modestate32] -> 32BitSelector38/1(x), 32BitSelector13/1(x)
  [modestate32] -> 32BitSelector39/1(x), 32BitSelector14/1(x)
  [modestate32] -> 32BitSelector15/1(x)
  [modestate32] -> 32BitSelector16/1(x)
  [modestate32] -> 32BitSelector17/1(x)
  [modestate32] -> 32BitSelector18/1(x)
  [modestate32] -> 32BitSelector19/1(x)
  [modestate32] -> 32BitSelector20/1(x)
  [modestate32] -> 32BitSelector21/1(x)
  [modestate32] -> 32BitSelector22/1(x)
  [modestate32] -> 32BitSelector23/1(x)
  [modestate32] -> 32BitSelector24/1(x)
  [modestate32] -> 32BitSelector25/1(x)
  RecvR4sMdDone_Val_read/1 -> Switch29/1
  RecvL4sMdDone_Val_read/1 -> Switch27/1
  [is4s] -> Switch27/2
  [is4s] -> Switch29/2
  [modestate32] -> 32BitSelector/1(x)
  Subsystem/1(MdDoneOut) -> [Md1Done]
  32BitSelector/1(y) -> Subsystem/2(MdEn)
  Subsystem1/1(MdDoneOut) -> [Md4Done]
  32BitSelector3/1(y) -> Subsystem1/2(MdEn)
  EZQMdDone_Val_read/1 -> Subsystem1/1(MdDone)
  Subsystem2/1(MdDoneOut) -> [Md5Done]
  32BitSelector4/1(y) -> Subsystem2/2(MdEn)
  INTMLMdDone_Val_read/1 -> Subsystem2/1(MdDone)
  Subsystem3/1(MdDoneOut) -> [Md6Done]
  32BitSelector5/1(y) -> Subsystem3/2(MdEn)
  32BitSelector6/1(y) -> Subsystem4/2(MdEn)
  Subsystem5/1(MdDoneOut) -> [Md8Done]
  Subsystem6/1(MdDoneOut) -> [Md9Done]
  Subsystem7/1(MdDoneOut) -> Data Type Conversion/1
  Subsystem8/1(MdDoneOut) -> Data Type Conversion1/1
  32BitSelector10/1(y) -> Subsystem8/2(MdEn)
  Subsystem9/1(MdDoneOut) -> Data Type Conversion2/1
  Subsystem10/1(MdDoneOut) -> Data Type Conversion3/1
  32BitSelector12/1(y) -> Subsystem10/2(MdEn)
  Subsystem11/1(MdDoneOut) -> [Md14Done]
  Subsystem12/1(MdDoneOut) -> [Md15Done]
  Subsystem13/1(MdDoneOut) -> [Md16Done]
  LgrstOpnLMdDone_Val_read/1 -> Subsystem13/1(MdDone)
  32BitSelector15/1(y) -> Subsystem13/2(MdEn)
  32BitSelector16/1(y) -> Subsystem14/2(MdEn)
  Subsystem14/1(MdDoneOut) -> [Md17Done]
  LgrstClsLMdDone_Val_read/1 -> Subsystem14/1(MdDone)
  32BitSelector17/1(y) -> Subsystem15/2(MdEn)
  LgrstOpnRMdDone_Val_read/1 -> Subsystem15/1(MdDone)
  Subsystem16/1(MdDoneOut) -> [Md19Done]
  LgrstClsRMdDone_Val_read/1 -> Subsystem16/1(MdDone)
  32BitSelector18/1(y) -> Subsystem16/2(MdEn)
  Subsystem17/1(MdDoneOut) -> [Md20Done]
  INTMRMdDone_Val_read/1 -> Subsystem17/1(MdDone)
  32BitSelector19/1(y) -> Subsystem17/2(MdEn)
  Subsystem18/1(MdDoneOut) -> [Md21Done]
  32BitSelector20/1(y) -> Subsystem18/2(MdEn)
  EZE4sLMdDone_Val_read/1 -> Subsystem18/1(MdDone)
  Subsystem19/1(MdDoneOut) -> [Md22Done]
  32BitSelector21/1(y) -> Subsystem19/2(MdEn)
  Subsystem20/1(MdDoneOut) -> [Md23Done]
  32BitSelector22/1(y) -> Subsystem20/2(MdEn)
  32BitSelector23/1(y) -> Subsystem21/2(MdEn)
  EZQ4sRMdDone_Val_read/1 -> Subsystem21/1(MdDone)
  Subsystem21/1(MdDoneOut) -> [Md24Done]
  32BitSelector24/1(y) -> Subsystem22/2(MdEn)
  Subsystem22/1(MdDoneOut) -> [Md25Done]
  32BitSelector25/1(y) -> Subsystem23/2(MdEn)
  WelcomeFwdMdDone_Val_read/1 -> Subsystem23/1(MdDone)
  Subsystem23/1(MdDoneOut) -> [Md26Done]
  Data Type Conversion/1 -> [Md10Done]
  Data Type Conversion1/1 -> [Md11Done]
  Data Type Conversion2/1 -> [Md12Done]
  Data Type Conversion3/1 -> [Md13Done]
  Data Type Conversion4/1 -> MdXX_MdDoneArray_Val_write/1
  EZQ4sLMdDone_Val_read/1 -> Subsystem19/1(MdDone)
  EZE4sRMdDone_Val_read/1 -> Subsystem20/1(MdDone)
  EZEMdDone_Val_read/1 -> Terminator/1
  Switch27/1 -> Subsystem8/1(MdDone)
  Switch29/1 -> Subsystem10/1(MdDone)
  EZE5576sMdDone_Val_read/1 -> Switch1/1
  EZE557MdDone_Val_read/1 -> Switch1/3
  Switch1/1 -> Subsystem/1(MdDone)
  Subsystem24/1(MdDoneOut) -> [Md32Done]
  Md32MdDone_Val_read/1 -> Subsystem24/1(MdDone)
  32BitSelector1/1(y) -> Subsystem24/2(MdEn)
  [modestate32] -> 32BitSelector1/1(x)
  LugLMdDone_Val_read/1 -> Switch2/3
  LugRMdDone_Val_read/1 -> Switch3/3
  Subsystem26/1(MdDoneOut) -> [Md30Done]
  Md30MdDone_Val_read/1 -> Subsystem26/1(MdDone)
  32BitSelector26/1(y) -> Subsystem26/2(MdEn)
  [modestate32] -> 32BitSelector26/1(x)
  [modestate32] -> 32BitSelector27/1(x)
  32BitSelector27/1(y) -> Subsystem27/2(MdEn)
  Md31MdDone_Val_read/1 -> Subsystem27/1(MdDone)
  Subsystem27/1(MdDoneOut) -> [Md31Done]
  Subsystem28/1(MdDoneOut) -> [Md18Done]
  Md53MdDone_Val_read/1 -> Subsystem28/1(MdDone)
  32BitSelector28/1(y) -> Subsystem28/2(MdEn)
  [modestate32] -> 32BitSelector28/1(x)
  [modestate32] -> 32BitSelector34/1(x), 32BitSelector29/1(x)
  Subsystem29/1(MdDoneOut) -> [Md27Done]
  Subsystem30/1(MdDoneOut) -> [Md28Done]
  [modestate32] -> 32BitSelector35/1(x), 32BitSelector30/1(x)
  Subsystem15/1(MdDoneOut) -> Terminator5/1
  VIPLMdDone_Val_read/1 -> Terminator6/1
  VIPL4sMdDone_Val_read/1 -> Terminator7/1
  VIPRMdDone_Val_read/1 -> Terminator8/1
  VIPR4sMdDone_Val_read/1 -> Terminator9/1
  VIPL557MdDone_Val_read/1 -> Switch26/1
  VIPL557LTMdDone_Val_read/1 -> Switch26/3
  VIPR557LTMdDone_Val_read/1 -> Switch28/3
  VIPR557MdDone_Val_read/1 -> Switch28/1
  Switch2/1 -> Subsystem5/1(MdDone)
  LugL557MdDone_Val_read/1 -> Switch2/1
  [is7s] -> Switch2/2
  Switch3/1 -> Subsystem6/1(MdDone)
  LugR557MdDone_Val_read/1 -> Switch3/1
  [is7s] -> Switch3/2
  Logical Operator/1 -> Subsystem7/2(MdEn)
  32BitSelector9/1(y) -> Logical Operator/1
  32BitSelector2/1(y) -> Logical Operator/2
  Logical Operator1/1 -> Subsystem9/2(MdEn)
  32BitSelector11/1(y) -> Logical Operator1/1
  32BitSelector31/1(y) -> Logical Operator1/2
  Logical Operator2/1 -> Subsystem5/2(MdEn)
  32BitSelector7/1(y) -> Logical Operator2/1
  32BitSelector32/1(y) -> Logical Operator2/2
  Logical Operator3/1 -> Subsystem6/2(MdEn)
  32BitSelector8/1(y) -> Logical Operator3/1
  32BitSelector33/1(y) -> Logical Operator3/2
  [modestate32] -> 32BitSelector8/1(x), 32BitSelector33/1(x)
  Logical Operator4/1 -> Subsystem29/2(MdEn)
  32BitSelector29/1(y) -> Logical Operator4/1
  32BitSelector34/1(y) -> Logical Operator4/2
  Logical Operator5/1 -> Subsystem30/2(MdEn)
  32BitSelector30/1(y) -> Logical Operator5/1
  32BitSelector35/1(y) -> Logical Operator5/2
  WelcomeBkwdMdDone_Val_read/1 -> Terminator3/1
  Switch/1 -> Subsystem22/1(MdDone)
  [is7s] -> Switch/2
  Md56MdDone_Val_read/1 -> Switch/1
  Md566sMdDone_Val_read/1 -> Switch/3
  Md57MdDone_Val_read/1 -> Subsystem25/1(MdDone)
  Md58MdDone_Val_read/1 -> Subsystem31/1(MdDone)
  32BitSelector36/1(y) -> Subsystem25/2(MdEn)
  [modestate32] -> 32BitSelector36/1(x)
  [modestate32] -> 32BitSelector37/1(x)
  32BitSelector37/1(y) -> Subsystem31/2(MdEn)
  Subsystem25/1(MdDoneOut) -> [Md57Done]
  Subsystem31/1(MdDoneOut) -> [Md58Done]
  FamlyLMdDone_Val_read/1 -> Terminator_11/1
  FamlyRMdDone_Val_read/1 -> Terminator_12/1
  PA_KeSMSuVehicleModelConfig_Val/1 -> Compare To Constant/1
  Compare To Constant/1 -> Switch4/2
  Md61MdDone_Val_read/1 -> Switch4/1
  Switch4/1 -> Subsystem3/1(MdDone)
  FwdLMdDone_Val_read/1 -> Switch4/3
  Compare To Constant1/1 -> Switch5/2
  PA_KeSMSuVehicleModelConfig_Val1/1 -> Compare To Constant1/1
  Md62MdDone_Val_read/1 -> Switch5/1
  Switch5/1 -> Subsystem4/1(MdDone)
  FwdRMdDone_Val_read/1 -> Switch5/3
  VIPL3582MdDone_Val_read/1 -> ?
  Switch28/1 -> Subsystem9/1(MdDone)
  VIPLExit557MdDone_Val_read/1 -> Subsystem29/1(MdDone)
  VIPRExit557MdDone_Val_read/1 -> Subsystem30/1(MdDone)
  IfVeSMSbSecRwLtStCshnFrntUpwdDnwdMovConfig_Val_read/1 -> Logical Operator6/1
  PA_KeSMSuVehicleModelConfig_Val2/1 -> Compare To Constant2/1
  Compare To Constant2/1 -> Logical Operator6/2
  Logical Operator6/1 -> Switch26/2
  Switch26/1 -> Subsystem7/1(MdDone)
  Compare To Constant3/1 -> Logical Operator7/2
  PA_KeSMSuVehicleModelConfig_Val3/1 -> Compare To Constant3/1
  IfVeSMSbSecRwRtStCshnFrntUpwdDnwdMovConfig_Val_read/1 -> Logical Operator7/1
  Logical Operator7/1 -> Switch28/2
  Md27MdDone_Val_read/1 -> Subsystem11/1(MdDone)
  Md28MdDone_Val_read/1 -> Subsystem12/1(MdDone)
  32BitSelector13/1(y) -> Logical Operator8/1
  Logical Operator8/1 -> Subsystem11/2(MdEn)
  32BitSelector38/1(y) -> Logical Operator8/2
  32BitSelector39/1(y) -> Logical Operator9/2
  32BitSelector14/1(y) -> Logical Operator9/1
  Logical Operator9/1 -> Subsystem12/2(MdEn)
  ComfortMdRDone_Val_read/1 -> Switch29/3
  ComfortMdLDone_Val_read/1 -> Switch27/3

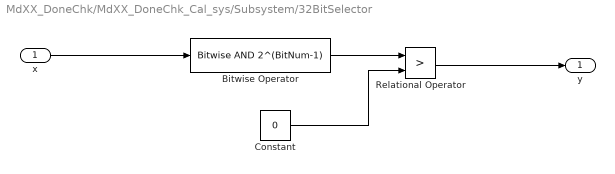
== system MdXX_DoneChk/MdXX_DoneChk_Cal_sys/Subsystem/32BitSelector ==
  x : Inport
  Bitwise Operator : simulink/Logic and Bit Operations/Bitwise Operator  logicop=AND  UseBitMask=on  BitMask=2^(BitNum-1)  BitMaskRealWorld=Stored Integer
  Constant : Constant  Value=0  OutDataTypeStr=uint32
  Relational Operator : RelationalOperator  Operator=>  OutDataTypeStr=boolean  RndMeth=Simplest  InputSameDT=off
  y : Outport  VectorParamsAs1DForOutWhenUnconnected=off
  wires:
  Relational Operator/1 -> y/1
  Constant/1 -> Relational Operator/2
  x/1 -> Bitwise Operator/1
  Bitwise Operator/1 -> Relational Operator/1

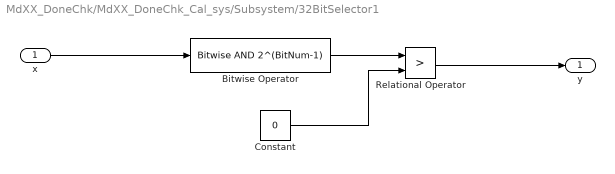
== system MdXX_DoneChk/MdXX_DoneChk_Cal_sys/Subsystem/32BitSelector1 ==
  x : Inport
  Bitwise Operator : simulink/Logic and Bit Operations/Bitwise Operator  logicop=AND  UseBitMask=on  BitMask=2^(BitNum-1)  BitMaskRealWorld=Stored Integer
  Constant : Constant  Value=0  OutDataTypeStr=uint32
  Relational Operator : RelationalOperator  Operator=>  OutDataTypeStr=boolean  RndMeth=Simplest  InputSameDT=off
  y : Outport  VectorParamsAs1DForOutWhenUnconnected=off
  wires:
  Relational Operator/1 -> y/1
  Constant/1 -> Relational Operator/2
  x/1 -> Bitwise Operator/1
  Bitwise Operator/1 -> Relational Operator/1

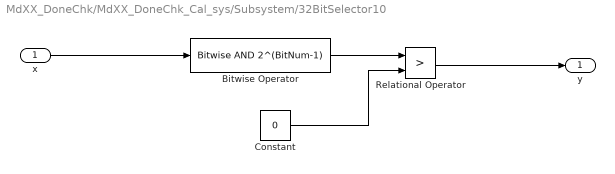
== system MdXX_DoneChk/MdXX_DoneChk_Cal_sys/Subsystem/32BitSelector10 ==
  x : Inport
  Bitwise Operator : simulink/Logic and Bit Operations/Bitwise Operator  logicop=AND  UseBitMask=on  BitMask=2^(BitNum-1)  BitMaskRealWorld=Stored Integer
  Constant : Constant  Value=0  OutDataTypeStr=uint32
  Relational Operator : RelationalOperator  Operator=>  OutDataTypeStr=boolean  RndMeth=Simplest  InputSameDT=off
  y : Outport  VectorParamsAs1DForOutWhenUnconnected=off
  wires:
  Relational Operator/1 -> y/1
  Constant/1 -> Relational Operator/2
  x/1 -> Bitwise Operator/1
  Bitwise Operator/1 -> Relational Operator/1

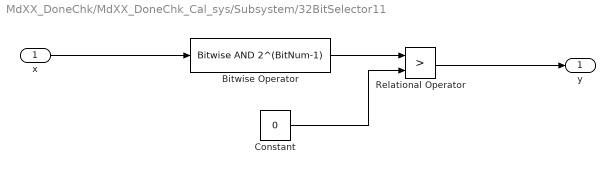
== system MdXX_DoneChk/MdXX_DoneChk_Cal_sys/Subsystem/32BitSelector11 ==
  x : Inport
  Bitwise Operator : simulink/Logic and Bit Operations/Bitwise Operator  logicop=AND  UseBitMask=on  BitMask=2^(BitNum-1)  BitMaskRealWorld=Stored Integer
  Constant : Constant  Value=0  OutDataTypeStr=uint32
  Relational Operator : RelationalOperator  Operator=>  OutDataTypeStr=boolean  RndMeth=Simplest  InputSameDT=off
  y : Outport  VectorParamsAs1DForOutWhenUnconnected=off
  wires:
  Bitwise Operator/1 -> Relational Operator/1
  x/1 -> Bitwise Operator/1
  Constant/1 -> Relational Operator/2
  Relational Operator/1 -> y/1

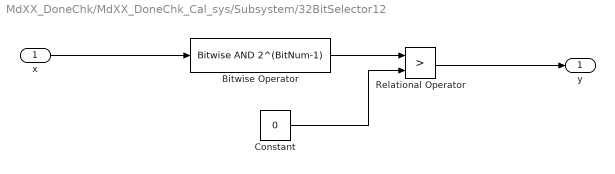
== system MdXX_DoneChk/MdXX_DoneChk_Cal_sys/Subsystem/32BitSelector12 ==
  x : Inport
  Bitwise Operator : simulink/Logic and Bit Operations/Bitwise Operator  logicop=AND  UseBitMask=on  BitMask=2^(BitNum-1)  BitMaskRealWorld=Stored Integer
  Constant : Constant  Value=0  OutDataTypeStr=uint32
  Relational Operator : RelationalOperator  Operator=>  OutDataTypeStr=boolean  RndMeth=Simplest  InputSameDT=off
  y : Outport  VectorParamsAs1DForOutWhenUnconnected=off
  wires:
  Relational Operator/1 -> y/1
  Constant/1 -> Relational Operator/2
  x/1 -> Bitwise Operator/1
  Bitwise Operator/1 -> Relational Operator/1

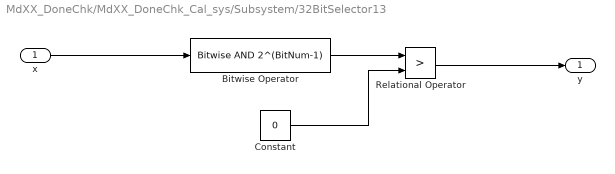
== system MdXX_DoneChk/MdXX_DoneChk_Cal_sys/Subsystem/32BitSelector13 ==
  x : Inport
  Bitwise Operator : simulink/Logic and Bit Operations/Bitwise Operator  logicop=AND  UseBitMask=on  BitMask=2^(BitNum-1)  BitMaskRealWorld=Stored Integer
  Constant : Constant  Value=0  OutDataTypeStr=uint32
  Relational Operator : RelationalOperator  Operator=>  OutDataTypeStr=boolean  RndMeth=Simplest  InputSameDT=off
  y : Outport  VectorParamsAs1DForOutWhenUnconnected=off
  wires:
  Bitwise Operator/1 -> Relational Operator/1
  x/1 -> Bitwise Operator/1
  Constant/1 -> Relational Operator/2
  Relational Operator/1 -> y/1
